simulink model "c09f12_01_avn"  (R2012b)
settings: Solver=ode45  StartTime=0.0  StopTime="(2^(7+2))  * (2^8)"  RelTol=1e-3
undefined symbols (not defined in the file): Down, pfb_coeff_gen_calc, Up, xlipgetpartsetting
libraries: xbsIndex_r4 x7041, casper_library_misc x193, xps_library x58, casper_library_delays x50, simulink x16, dspsigops x12, casper_library_flow_control x5, xbsReplacements_r4 x4, casper_library_ffts_twiddle x2, casper_library_multipliers x2, casper_library_reorder x1
(part 1 of 77)
settings Model: Creator=root  LastModifiedBy=brains
settings DataIOCC: LimitDataPoints=off  SignalLoggingSaveFormat=ModelDataLogs
settings DebuggingCC: FcnCallInpInsideContextMsg=UseLocalSettings  StrictBusMsg=Warning
settings GRTTargetCC: CombineOutputUpdateFcns=off  GRTInterface=on

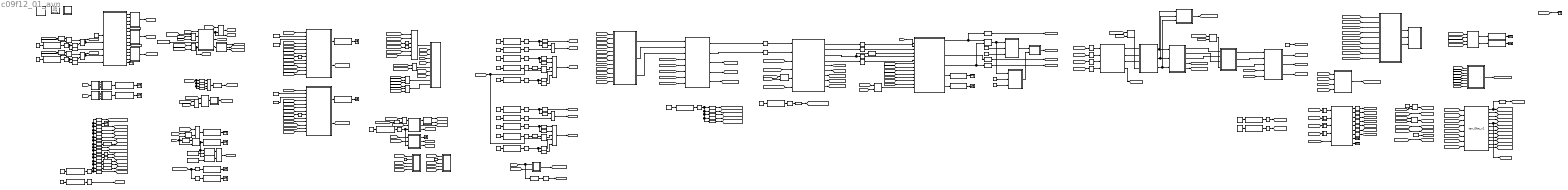
== system c09f12_01_avn ==
  note: Accept 32 data words from ibob,
      | plus a 1 word header,
      | creating UDP packets of length 33 x 64 bits.
      | This block generates the destination IP address.
  note: Data in: 18bits real only x 2
  note: RCS:
      |
      | 1. 04-08-2011
      | - Initial revision.
      | 2. 08-08-2011
      | - New snapshots for easier timing.
      | 3. 17-08-2011
      | - Fixed logic around gbe & xaui snaps.
      | 4. 19-08-2011
      | - Updated timing logic from latest wideband build.
      | ...
      | 5. 17-11-2011
      | - New TVG before CT.
      | - New DV gen in fine chan.
      | - Remove delay on sync in packetiser.
      |
      | New packetiser put in, builds, but 10Gbe doesn't
      | work. Why? If the device is too full?
      |
      | Needs coarse vector accumulator.
      |
      | 6. 10-01-2012
      | - 16 x-engines vs 4 seems to solve VACC overflow
      | on the x-engine.
      | 7. 12-01-2012
      | - Move to 4a 8x to for lab work.
      | - Also mux to bypass window before fine FFT.
      | 8. 18-01-2012
      | - Cleaned up fine snap
      | - Delays between blocks in coarse channelisaiton.
      | 9. 10-02-2012
      | - See subversion for notes.
      | 10. 13-02-2012
      | - Half of channel select in the coarse section,
      | moved from fine buffer.
      | - No more mixer, so real PFB and FFT.
  note: The data out of the QDR
      | ct is 64-bit data ready
      | for the packetiser.
  note: * A resync command will cause the sync_gen to stop issuing sync pulses.
      | * It will then ignore the next input trigger (1PPS), while sync is flushed through the DSP pipeline.
      | * It will then lock onto the next trigger (1PPS) and issue a sync.
      | * Need a multiple of (pfb_fir taps*LCM(FFT reorder orders) *fft bins/parallel inputs =)
      | (4 * LCM(2,2,2,9) * 2048 / 4) = 9216) for sync_period for simulation
  note: data alignment infrastructure to
      | align to within one clock cycle
      | using PPS
  note: clock and synchronisation
      | info
  note: Status registers
  note: LEDs
  note: delay tracking and
      | fringe stopping registers
  note: pol0
  note: pol1
  note: Fine delay tracking and
      | fringe stopping
  note: ADC snap blocks
  " System Generator" : xbsIndex_r4/ System Generator  Tag=genX  xilinxfamily=virtex5  part=xc5vsx95t  speed=-1  package=ff1136  synthesis_tool=XST  clock_wrapper=Clock Enables  directory=./c09f12_01_avn/sysgen  proj_type=Project Navigator  Synth_file=XST Defaults  Impl_file=ISE Defaults  testbench=off  simulink_period=1  sysclk_period=5  dcm_input_clock_period=100  incr_netlist=off  trim_vbits=Everywhere in SubSystem  dbl_ovrd=According to Block Masks  core_generation=According to Block Masks  run_coregen=off  deprecated_control=off  eval_field=0  block_type=sysgen
      settings: block_version=11.4
  AddSub : xbsIndex_r4/AddSub  mode=Addition  use_carryin=off  use_carryout=off  en=off  latency=1  precision=User Defined  arith_type=Unsigned  n_bits=15  bin_pt=0  quantization=Truncate  overflow=Saturate  dbl_ovrd=off  use_behavioral_HDL=off  hw_selection=DSP48  pipelined=on  block_type=addsub
  AddSub1 : xbsIndex_r4/AddSub  mode=Addition  use_carryin=off  use_carryout=off  en=off  latency=1  precision=User Defined  arith_type=Unsigned  n_bits=15  bin_pt=0  quantization=Truncate  overflow=Saturate  dbl_ovrd=off  use_behavioral_HDL=off  hw_selection=DSP48  pipelined=on  block_type=addsub
  Concat : xbsIndex_r4/Concat  num_inputs=3  dbl_ovrd=off  block_type=concat
      settings: block_version=10.1.3
  Concat1 : xbsIndex_r4/Concat  num_inputs=5  dbl_ovrd=off  block_type=concat
      settings: block_version=10.1.3
  Concat{2,6,9,21} (4 alike) : xbsIndex_r4/Concat  num_inputs=2  dbl_ovrd=off  block_type=concat
      Concat2 settings: block_version=10.1.3
      Concat9 settings: block_version=10.1.3
  Concat22 : xbsIndex_r4/Concat  num_inputs=5  dbl_ovrd=off  block_type=concat
      settings: block_version=10.1.3
  Constant : Constant  SampleTime=1/4
  Constant{1,6,9,11,18,27,33,48} (8 alike) : Constant  Value=0
  Constant{10,13,16,21..22,32} (6 alike) : Constant  Value=8
  Constant14 : xbsIndex_r4/Constant  const=1  gui_display_data_type=Fixed-point  arith_type=Boolean  n_bits=1  bin_pt=0  preci_type=Single  exp_width=8  frac_width=24  explicit_period=on  period=1  equ=P=C  opselect=C  inp2=PCIN>>17  opr=+  inp1=P  carry=CIN  dbl_ovrd=off  block_type=constant
  Constant15 : xbsIndex_r4/Constant  const=1  gui_display_data_type=Fixed-point  arith_type=Boolean  n_bits=1  bin_pt=0  preci_type=Single  exp_width=8  frac_width=24  explicit_period=off  period=1  equ=P=C  opselect=C  inp2=PCIN>>17  opr=+  inp1=P  carry=CIN  dbl_ovrd=off  block_type=constant
      settings: block_version=11.4
  Constant17 : xbsIndex_r4/Constant  const=0  gui_display_data_type=Fixed-point  arith_type=Boolean  n_bits=16  bin_pt=14  preci_type=Single  exp_width=8  frac_width=24  explicit_period=on  period=1  equ=P=C  opselect=C  inp2=PCIN>>17  opr=+  inp1=P  carry=CIN  dbl_ovrd=off  block_type=constant
      settings: block_version=11.4
  Constant20 : xbsIndex_r4/Constant  const=0  gui_display_data_type=Fixed-point  arith_type=Boolean  n_bits=1  bin_pt=0  preci_type=Single  exp_width=8  frac_width=24  explicit_period=on  period=1  equ=P=C  opselect=C  inp2=PCIN>>17  opr=+  inp1=P  carry=CIN  dbl_ovrd=off  block_type=constant
      settings: block_version=11.3
  Constant23 : xbsIndex_r4/Constant  const=1  gui_display_data_type=Fixed-point  arith_type=Boolean  n_bits=1  bin_pt=0  preci_type=Single  exp_width=8  frac_width=24  explicit_period=off  period=1  equ=P=C  opselect=C  inp2=PCIN>>17  opr=+  inp1=P  carry=CIN  dbl_ovrd=off  block_type=constant
      settings: block_version=11.4
  Constant24 : xbsIndex_r4/Constant  const=0  gui_display_data_type=Fixed-point  arith_type=Boolean  n_bits=64  bin_pt=0  preci_type=Single  exp_width=8  frac_width=24  explicit_period=off  period=1  equ=P=C  opselect=C  inp2=PCIN>>17  opr=+  inp1=P  carry=CIN  dbl_ovrd=off  block_type=constant
      settings: block_version=11.4
  Constant25 : Constant  Value=100
  Constant29 : Constant  Value=20
  Constant37 : xbsIndex_r4/Constant  const=800000000/4-1  gui_display_data_type=Fixed-point  arith_type=Unsigned  n_bits=32  bin_pt=0  preci_type=Single  exp_width=8  frac_width=24  explicit_period=on  period=1  equ=P=C  opselect=C  inp2=PCIN>>17  opr=+  inp1=P  carry=CIN  dbl_ovrd=off  block_type=constant
      settings: block_version=11.4
  Constant41 : xbsIndex_r4/Constant  const=0  gui_display_data_type=Fixed-point  arith_type=Unsigned  n_bits=32  bin_pt=0  preci_type=Single  exp_width=8  frac_width=24  explicit_period=off  period=1  equ=P=C  opselect=C  inp2=PCIN>>17  opr=+  inp1=P  carry=CIN  dbl_ovrd=off  block_type=constant
      settings: block_version=11.4
  Constant46 : xbsIndex_r4/Constant  const=0  gui_display_data_type=Fixed-point  arith_type=Boolean  n_bits=64  bin_pt=0  preci_type=Single  exp_width=8  frac_width=24  explicit_period=off  period=1  equ=P=C  opselect=C  inp2=PCIN>>17  opr=+  inp1=P  carry=CIN  dbl_ovrd=off  block_type=constant
      settings: block_version=11.4
  Constant5 : xbsIndex_r4/Constant  const=800000000/4+1  gui_display_data_type=Fixed-point  arith_type=Unsigned  n_bits=32  bin_pt=0  preci_type=Single  exp_width=8  frac_width=24  explicit_period=on  period=1  equ=P=C  opselect=C  inp2=PCIN>>17  opr=+  inp1=P  carry=CIN  dbl_ovrd=off  block_type=constant
      settings: block_version=11.4
  Constant7 : Constant  Value=20
  Constant8 : xbsIndex_r4/Constant  const=0  gui_display_data_type=Fixed-point  arith_type=Unsigned  n_bits=32  bin_pt=0  preci_type=Single  exp_width=8  frac_width=24  explicit_period=off  period=1  equ=P=C  opselect=C  inp2=PCIN>>17  opr=+  inp1=P  carry=CIN  dbl_ovrd=off  block_type=constant
      settings: block_version=11.4
  Counter1 : xbsIndex_r4/Counter  cnt_type=Free Running  cnt_to=Inf  operation=Up  start_count=1  cnt_by_val=1  arith_type=Unsigned  n_bits=32  bin_pt=0  load_pin=off  rst=on  en=off  explicit_period=on  period=1  dbl_ovrd=off  use_behavioral_HDL=off  implementation=Fabric  use_rpm=on  block_type=counter
  Counter3 : xbsIndex_r4/Counter  cnt_type=Free Running  cnt_to=Inf  operation=Up  start_count=0  cnt_by_val=1  arith_type=Unsigned  n_bits=31  bin_pt=0  load_pin=off  rst=on  en=on  explicit_period=on  period=1  dbl_ovrd=off  use_behavioral_HDL=off  implementation=DSP48  use_rpm=on  block_type=counter
  Counter8 : xbsIndex_r4/Counter  cnt_type=Free Running  cnt_to=Inf  operation=Up  start_count=0  cnt_by_val=1  arith_type=Unsigned  n_bits=12  bin_pt=0  load_pin=off  rst=on  en=on  explicit_period=on  period=1  dbl_ovrd=off  use_behavioral_HDL=off  implementation=Fabric  block_type=counter
      settings: block_version=11.4
  Delay{1,8,12..22,24..30,32,35..37,39..46} (32 alike) : xbsIndex_r4/Delay  rst=off  infoeditControl=Selection of Reset will increase slice count due to use of real FFs and instead of SRLs  en=off  latency=1  dbl_ovrd=off  reg_retiming=on  block_type=delay
      Delay13 settings: block_version=11.4
      Delay14 settings: block_version=11.4
      Delay15 settings: block_version=11.4
      Delay16 settings: block_version=11.4
      Delay17 settings: block_version=11.4
      Delay18 settings: block_version=11.4
      Delay19 settings: block_version=11.4
      Delay20 settings: block_version=11.4
      Delay21 settings: block_version=11.4
      Delay22 settings: block_version=11.4
      Delay24 settings: block_version=11.4
      Delay25 settings: block_version=11.4
      Delay26 settings: block_version=11.4
      Delay27 settings: block_version=11.4
      Delay28 settings: block_version=11.4
      Delay29 settings: block_version=11.4
      Delay30 settings: block_version=11.4
      Delay32 settings: block_version=11.4
      Delay35 settings: block_version=11.4
      Delay36 settings: block_version=11.4
      Delay37 settings: block_version=11.4
      Delay39 settings: block_version=11.4
      Delay40 settings: block_version=11.4
      Delay41 settings: block_version=11.4
      Delay42 settings: block_version=11.4
  Delay10 : Subsystem  AncestorBlock=casper_library/Delays/pipeline  mask(pipeline){latency=1}
      mask help:
      | An explicitly laid-out delay line to avoid mapping to SRL16s
      | for use in pipelining to help achieve timing closure.
      mask init:
      | pipeline_init(gcb, 'latency', latency);
      mask Display:
      | port_label('input', 1, 'd');
      | port_label('output', 1, 'q');
      | disp(['Z^-', num2str(latency)]);
  Delay100 : Subsystem  AncestorBlock=casper_library/Delays/pipeline  mask(pipeline){latency=2}
      mask help:
      | An explicitly laid-out delay line to avoid mapping to SRL16s
      | for use in pipelining to help achieve timing closure.
      mask init:
      | pipeline_init(gcb, 'latency', latency);
      mask Display:
      | port_label('input', 1, 'd');
      | port_label('output', 1, 'q');
      | disp(['Z^-', num2str(latency)]);
  Delay11 : Subsystem  AncestorBlock=casper_library/Delays/pipeline  mask(pipeline){latency=1}
      mask help:
      | An explicitly laid-out delay line to avoid mapping to SRL16s
      | for use in pipelining to help achieve timing closure.
      mask init:
      | pipeline_init(gcb, 'latency', latency);
      mask Display:
      | port_label('input', 1, 'd');
      | port_label('output', 1, 'q');
      | disp(['Z^-', num2str(latency)]);
  Delay2 : Subsystem  AncestorBlock=casper_library/Delays/pipeline  mask(pipeline){latency=2}
      mask help:
      | An explicitly laid-out delay line to avoid mapping to SRL16s
      | for use in pipelining to help achieve timing closure.
      mask init:
      | pipeline_init(gcb, 'latency', latency);
      mask Display:
      | port_label('input', 1, 'd');
      | port_label('output', 1, 'q');
      | disp(['Z^-', num2str(latency)]);
  Delay23 : Subsystem  AncestorBlock=casper_library/Delays/pipeline  mask(pipeline){latency=1}
      mask help:
      | An explicitly laid-out delay line to avoid mapping to SRL16s
      | for use in pipelining to help achieve timing closure.
      mask init:
      | pipeline_init(gcb, 'latency', latency);
      mask Display:
      | port_label('input', 1, 'd');
      | port_label('output', 1, 'q');
      | disp(['Z^-', num2str(latency)]);
  Delay3 : Subsystem  AncestorBlock=casper_library/Delays/pipeline  mask(pipeline){latency=1}
      mask help:
      | An explicitly laid-out delay line to avoid mapping to SRL16s
      | for use in pipelining to help achieve timing closure.
      mask init:
      | pipeline_init(gcb, 'latency', latency);
      mask Display:
      | port_label('input', 1, 'd');
      | port_label('output', 1, 'q');
      | disp(['Z^-', num2str(latency)]);
  Delay31 : Subsystem  AncestorBlock=casper_library/Delays/pipeline  mask(pipeline){latency=1}
      mask help:
      | An explicitly laid-out delay line to avoid mapping to SRL16s
      | for use in pipelining to help achieve timing closure.
      mask init:
      | pipeline_init(gcb, 'latency', latency);
      mask Display:
      | port_label('input', 1, 'd');
      | port_label('output', 1, 'q');
      | disp(['Z^-', num2str(latency)]);
  Delay33 : Subsystem  AncestorBlock=casper_library/Delays/pipeline  mask(pipeline){latency=1}
      mask help:
      | An explicitly laid-out delay line to avoid mapping to SRL16s
      | for use in pipelining to help achieve timing closure.
      mask init:
      | pipeline_init(gcb, 'latency', latency);
      mask Display:
      | port_label('input', 1, 'd');
      | port_label('output', 1, 'q');
      | disp(['Z^-', num2str(latency)]);
  Delay34 : Subsystem  AncestorBlock=casper_library/Delays/pipeline  mask(pipeline){latency=1}
      mask help:
      | An explicitly laid-out delay line to avoid mapping to SRL16s
      | for use in pipelining to help achieve timing closure.
      mask init:
      | pipeline_init(gcb, 'latency', latency);
      mask Display:
      | port_label('input', 1, 'd');
      | port_label('output', 1, 'q');
      | disp(['Z^-', num2str(latency)]);
  Delay4 : Subsystem  AncestorBlock=casper_library/Delays/pipeline  mask(pipeline){latency=1}
      mask help:
      | An explicitly laid-out delay line to avoid mapping to SRL16s
      | for use in pipelining to help achieve timing closure.
      mask init:
      | pipeline_init(gcb, 'latency', latency);
      mask Display:
      | port_label('input', 1, 'd');
      | port_label('output', 1, 'q');
      | disp(['Z^-', num2str(latency)]);
  Delay5 : Subsystem  AncestorBlock=casper_library/Delays/pipeline  mask(pipeline){latency=1}
      mask help:
      | An explicitly laid-out delay line to avoid mapping to SRL16s
      | for use in pipelining to help achieve timing closure.
      mask init:
      | pipeline_init(gcb, 'latency', latency);
      mask Display:
      | port_label('input', 1, 'd');
      | port_label('output', 1, 'q');
      | disp(['Z^-', num2str(latency)]);
  Delay6 : xbsIndex_r4/Delay  rst=off  infoeditControl=Selection of Reset will increase slice count due to use of real FFs and instead of SRLs  en=off  latency=1  dbl_ovrd=off  reg_retiming=off  block_type=delay
      settings: block_version=11.4
  Delay7 : Subsystem  AncestorBlock=casper_library/Delays/pipeline  mask(pipeline){latency=1}
      mask help:
      | An explicitly laid-out delay line to avoid mapping to SRL16s
      | for use in pipelining to help achieve timing closure.
      mask init:
      | pipeline_init(gcb, 'latency', latency);
      mask Display:
      | port_label('input', 1, 'd');
      | port_label('output', 1, 'q');
      | disp(['Z^-', num2str(latency)]);
  Delay9 : Subsystem  AncestorBlock=casper_library/Delays/pipeline  mask(pipeline){latency=1}
      mask help:
      | An explicitly laid-out delay line to avoid mapping to SRL16s
      | for use in pipelining to help achieve timing closure.
      mask init:
      | pipeline_init(gcb, 'latency', latency);
      mask Display:
      | port_label('input', 1, 'd');
      | port_label('output', 1, 'q');
      | disp(['Z^-', num2str(latency)]);
  Inverter{,1..6} (7 alike) : xbsIndex_r4/Inverter  en=off  latency=0  dbl_ovrd=off  block_type=inv
      settings: block_version=11.4
  Logical1 : xbsIndex_r4/Logical  logical_function=OR  inputs=4  en=off  latency=0  precision=Full  arith_type=Unsigned  n_bits=16  bin_pt=0  align_bp=on  dbl_ovrd=off  block_type=logical
  Logical10 : xbsIndex_r4/Logical  logical_function=AND  inputs=2  en=off  latency=0  precision=Full  arith_type=Unsigned  n_bits=16  bin_pt=0  align_bp=on  dbl_ovrd=off  block_type=logical
  Logical11 : xbsIndex_r4/Logical  logical_function=AND  inputs=2  en=off  latency=0  precision=Full  arith_type=Unsigned  n_bits=16  bin_pt=0  align_bp=on  dbl_ovrd=off  block_type=logical
  Logical12 : xbsIndex_r4/Logical  logical_function=OR  inputs=3  en=off  latency=1  precision=Full  arith_type=Unsigned  n_bits=16  bin_pt=0  align_bp=on  dbl_ovrd=off  block_type=logical
  Logical{5..6,9,14,21} (5 alike) : xbsIndex_r4/Logical  logical_function=OR  inputs=2  en=off  latency=0  precision=Full  arith_type=Unsigned  n_bits=16  bin_pt=0  align_bp=on  dbl_ovrd=off  block_type=logical
      Logical21 settings: block_version=11.4
  Logical17 : xbsIndex_r4/Logical  logical_function=OR  inputs=3  en=off  latency=1  precision=Full  arith_type=Unsigned  n_bits=16  bin_pt=0  align_bp=on  dbl_ovrd=off  block_type=logical
  Logical2 : xbsIndex_r4/Logical  logical_function=AND  inputs=2  en=off  latency=0  precision=Full  arith_type=Unsigned  n_bits=8  bin_pt=2  align_bp=on  dbl_ovrd=off  block_type=logical
      settings: xl_area=[0, 0, 0, 0, 0, 0, 0]
  Logical3 : xbsIndex_r4/Logical  logical_function=OR  inputs=2  en=off  latency=1  precision=Full  arith_type=Unsigned  n_bits=8  bin_pt=2  align_bp=on  dbl_ovrd=off  block_type=logical
      settings: xl_area=[0, 0, 0, 0, 0, 0, 0]
  Logical4 : xbsIndex_r4/Logical  logical_function=OR  inputs=2  en=off  latency=1  precision=Full  arith_type=Unsigned  n_bits=16  bin_pt=0  align_bp=on  dbl_ovrd=off  block_type=logical
  Logical7 : xbsIndex_r4/Logical  logical_function=OR  inputs=6  en=off  latency=1  precision=Full  arith_type=Unsigned  n_bits=16  bin_pt=0  align_bp=on  dbl_ovrd=off  block_type=logical
  Logical8 : xbsIndex_r4/Logical  logical_function=AND  inputs=2  en=off  latency=0  precision=Full  arith_type=Unsigned  n_bits=16  bin_pt=0  align_bp=on  dbl_ovrd=off  block_type=logical
  Register{1..5,19} (6 alike) : xbsIndex_r4/Register  init=0  rst=off  en=on  dbl_ovrd=off  block_type=register
      Register1 settings: block_version=11.4
      Register2 settings: block_version=11.4
      Register3 settings: block_version=11.4
      Register4 settings: block_version=11.4
      Register5 settings: block_version=11.4
  Relational : xbsIndex_r4/Relational  mode=a>b  en=off  latency=1  dbl_ovrd=off  block_type=relational
  Relational1 : xbsIndex_r4/Relational  mode=a<b  en=off  latency=1  dbl_ovrd=off  block_type=relational
  Slice : xbsIndex_r4/Slice  nbits=32  boolean_output=off  mode=Lower Bit Location + Width  bit1=0  base1=MSB of Input  bit0=0  base0=LSB of Input  dbl_ovrd=off  block_type=slice
  Slice{1..2,4,12,15,73} (6 alike) : xbsIndex_r4/Slice  nbits=16  boolean_output=off  mode=Lower Bit Location + Width  bit1=0  base1=MSB of Input  bit0=0  base0=LSB of Input  dbl_ovrd=off  block_type=slice
      settings: infoedit="Extracts a given range of bits from each input sample and presents it at the output.  The output type is ordinarily unsigned with binary point at zero, but can be Boolean when the slice is one bit wide.<P><P>Hardware notes: In hardware this block costs nothing."  block_version=10.1.3
  Slice{3,7..8,10} (4 alike) : xbsIndex_r4/Slice  nbits=16  boolean_output=off  mode=Lower Bit Location + Width  bit1=0  base1=MSB of Input  bit0=16  base0=LSB of Input  dbl_ovrd=off  block_type=slice
      Slice10 settings: block_version=10.1.3
      Slice3 settings: infoedit="Extracts a given range of bits from each input sample and presents it at the output.  The output type is ordinarily unsigned with binary point at zero, but can be Boolean when the slice is one bit wide.<P><P>Hardware notes: In hardware this block costs nothing."  block_version=10.1.3
      Slice7 settings: block_version=10.1.3
      Slice8 settings: infoedit="Extracts a given range of bits from each input sample and presents it at the output.  The output type is ordinarily unsigned with binary point at zero, but can be Boolean when the slice is one bit wide.<P><P>Hardware notes: In hardware this block costs nothing."  block_version=10.1.3
  Slice{11,13,29,33} (4 alike) : xbsIndex_r4/Slice  nbits=1  boolean_output=on  mode=Upper Bit Location + Width  bit1=0  base1=MSB of Input  bit0=0  base0=LSB of Input  dbl_ovrd=off  block_type=slice
      Slice11 settings: block_version=10.1.3
      Slice13 settings: block_version=10.1.3
  Slice14 : xbsIndex_r4/Slice  nbits=15  boolean_output=off  mode=Lower Bit Location + Width  bit1=0  base1=MSB of Input  bit0=0  base0=LSB of Input  dbl_ovrd=off  block_type=slice
      settings: block_version=10.1.3
  Slice16 : xbsIndex_r4/Slice  nbits=32  boolean_output=off  mode=Lower Bit Location + Width  bit1=0  base1=MSB of Input  bit0=0  base0=LSB of Input  dbl_ovrd=off  block_type=slice
  Slice17 : xbsIndex_r4/Slice  nbits=1  boolean_output=on  mode=Lower Bit Location + Width  bit1=0  base1=MSB of Input  bit0=20  base0=LSB of Input  dbl_ovrd=off  block_type=slice
      settings: block_version=10.1.3
  Slice18 : xbsIndex_r4/Slice  nbits=1  boolean_output=on  mode=Lower Bit Location + Width  bit1=0  base1=MSB of Input  bit0=21  base0=LSB of Input  dbl_ovrd=off  block_type=slice
      settings: block_version=10.1.3
  Slice19 : xbsIndex_r4/Slice  nbits=8 - 1 - 1  boolean_output=off  mode=Lower Bit Location + Width  bit1=0  base1=MSB of Input  bit0=22  base0=LSB of Input  dbl_ovrd=off  block_type=slice
      settings: block_version=10.1.3
  Slice21 : xbsIndex_r4/Slice  nbits=10  boolean_output=off  mode=Lower Bit Location + Width  bit1=0  base1=MSB of Input  bit0=10  base0=LSB of Input  dbl_ovrd=off  block_type=slice
      settings: block_version=10.1.3
  Slice24 : xbsIndex_r4/Slice  nbits=26  boolean_output=off  mode=Lower Bit Location + Width  bit1=0  base1=MSB of Input  bit0=0  base0=LSB of Input  dbl_ovrd=off  block_type=slice
      settings: block_version=10.1.3
  Slice30 : xbsIndex_r4/Slice  nbits=6  boolean_output=off  mode=Lower Bit Location + Width  bit1=0  base1=MSB of Input  bit0=0  base0=LSB of Input  dbl_ovrd=off  block_type=slice
  Slice34 : xbsIndex_r4/Slice  nbits=6  boolean_output=off  mode=Lower Bit Location + Width  bit1=0  base1=MSB of Input  bit0=0  base0=LSB of Input  dbl_ovrd=off  block_type=slice
  Slice35 : xbsIndex_r4/Slice  nbits=1  boolean_output=on  mode=Lower Bit Location + Width  bit1=0  base1=MSB of Input  bit0=3  base0=LSB of Input  dbl_ovrd=off  block_type=slice
  Slice36 : xbsIndex_r4/Slice  nbits=1  boolean_output=on  mode=Lower Bit Location + Width  bit1=0  base1=MSB of Input  bit0=2  base0=LSB of Input  dbl_ovrd=off  block_type=slice
  Slice38 : xbsIndex_r4/Slice  nbits=15  boolean_output=off  mode=Lower Bit Location + Width  bit1=0  base1=MSB of Input  bit0=0  base0=LSB of Input  dbl_ovrd=off  block_type=slice
      settings: block_version=10.1.3
  Slice40 : xbsIndex_r4/Slice  nbits=1  boolean_output=on  mode=Lower Bit Location + Width  bit1=0  base1=MSB of Input  bit0=1  base0=LSB of Input  dbl_ovrd=off  block_type=slice
  Slice45 : xbsIndex_r4/Slice  nbits=1  boolean_output=on  mode=Lower Bit Location + Width  bit1=0  base1=MSB of Input  bit0=0  base0=LSB of Input  dbl_ovrd=off  block_type=slice
  Slice6 : xbsIndex_r4/Slice  nbits=10  boolean_output=off  mode=Lower Bit Location + Width  bit1=0  base1=MSB of Input  bit0=0  base0=LSB of Input  dbl_ovrd=off  block_type=slice
      settings: block_version=10.1.3
  Slice78 : xbsIndex_r4/Slice  nbits=1  boolean_output=on  mode=Lower Bit Location + Width  bit1=0  base1=MSB of Input  bit0=0  base0=LSB of Input  dbl_ovrd=off  block_type=slice
      settings: block_version=10.1.3
  Slice9 : xbsIndex_r4/Slice  nbits=32  boolean_output=off  mode=Lower Bit Location + Width  bit1=0  base1=MSB of Input  bit0=32  base0=LSB of Input  dbl_ovrd=off  block_type=slice
  Subsystem : Subsystem
  Subsystem1 : Subsystem
  Subsystem2 : Subsystem
  Subsystem3 : Subsystem
  Subsystem4 : Subsystem
  Terminator{,1..15,17,25} (18 alike) : Terminator
  XSG core config : xps_library/XSG core config  Tag=xps:xsg  hw_sys=ROACH:sx95t  clk_src=adc0_clk  ROACH_clk_src=adc0_clk  ROACH2_clk_src=adc0_clk  clk_rate=800/4  sample_period=1  synthesis_tool=XST
  a0_fd0 : xps_library/software register  Tag=xps:sw_reg  io_dir=From Processor  arith_type=Unsigned  bitwidth=32  bin_pt=0  sample_period=1  gw_name=c09f12_01_avn_a0_fd0_user_data_out
      link override c09f12_01_a0_fd0_user_data_out: arith_type=Unsigned  n_bits=32  bin_pt=0  period=1
  a0_fd1 : xps_library/software register  Tag=xps:sw_reg  io_dir=From Processor  arith_type=Unsigned  bitwidth=32  bin_pt=0  sample_period=1  gw_name=c09f12_01_avn_a0_fd1_user_data_out
      link override c09f12_01_a0_fd1_user_data_out: arith_type=Unsigned  n_bits=32  bin_pt=0  period=1
  a1_fd0 : xps_library/software register  Tag=xps:sw_reg  io_dir=From Processor  arith_type=Unsigned  bitwidth=32  bin_pt=0  sample_period=1  gw_name=c09f12_01_avn_a1_fd0_user_data_out
      link override c09f12_01_a1_fd0_user_data_out: arith_type=Unsigned  n_bits=32  bin_pt=0  period=1
  a1_fd1 : xps_library/software register  Tag=xps:sw_reg  io_dir=From Processor  arith_type=Unsigned  bitwidth=32  bin_pt=0  sample_period=1  gw_name=c09f12_01_avn_a1_fd1_user_data_out
      link override c09f12_01_a1_fd1_user_data_out: arith_type=Unsigned  n_bits=32  bin_pt=0  period=1
  adc_ctrl0 : xps_library/software register  Tag=xps:sw_reg  io_dir=From Processor  arith_type=Unsigned  bitwidth=32  bin_pt=0  sample_period=1  gw_name=c09f12_01_avn_adc_ctrl0_user_data_out
      link override c09f12_01_adc_ctrl0_user_data_out: arith_type=Unsigned  n_bits=32  bin_pt=0  period=1
  adc_ctrl1 : xps_library/software register  Tag=xps:sw_reg  io_dir=From Processor  arith_type=Unsigned  bitwidth=32  bin_pt=0  sample_period=1  gw_name=c09f12_01_avn_adc_ctrl1_user_data_out
      link override c09f12_01_adc_ctrl1_user_data_out: arith_type=Unsigned  n_bits=32  bin_pt=0  period=1
  adc_snap0 : Subsystem  mask(snapshot){storage=bram, dram_dimm=1, dram_clock=200, nsamples=10, data_width=32, offset=on, circap=on, value=on, use_dsp48=off}
      mask prompts: storage "Storage medium"; dram_dimm "DRAM dimm"; dram_clock "DRAM clock rate"; nsamples "Number of Samples (2^?)"; data_width "Data width"; offset "Start delay support"; circap "Circular capture support"; value "Extra value capture support"; use_dsp48 "Use DSP48s to implement counters"
      mask help:
      | Standard snap block, but with the following optional extras;
      |  1) Optionally delay the fabric trigger by a user-specified number of valids.
      |  2) Capture continuously after a trigger until a stop pulse is received. Data is captured into BRAM continuously, with old data being overwritten until a stop command is received. Then stop capturing when memory is filled. This enables you to get some data before and some data after the stop pulse. Use the 'tr_en_cnt' register to determine where you are in your vector. 'Addr' register's MSb now indicates 'busy capturing'.
      |  3) Optionally capture a value on an input port to a register at the same time as the first data sample.
      |  4) Implement counters using DSP48Es to save resources.
      mask init:
      | snapshot_init(gcb, ...
      |     'storage', storage, ...
      |     'dram_dimm', dram_dimm, ...
      |     'dram_clock', dram_clock, ...
      |     'nsamples', nsamples, ...
      |     'data_width', data_width, ...
      |     'offset', offset, ...
      |     'circap', circap, ...
      |     'value', value, ...
      |     'use_dsp48', use_dsp48);
      mask TypeOptions storage: bram | dram
      mask Callback storage: snapshot_callback();
      mask TypeOptions dram_dimm: 1 | 2 | 3 | 4
      mask TypeOptions dram_clock: 200 | 250 | 266 | 300 | 333
      mask TypeOptions data_width: 8 | 16 | 32 | 64 | 128
  adc_snap1 : Subsystem  mask(snapshot){storage=bram, dram_dimm=1, dram_clock=200, nsamples=10, data_width=32, offset=on, circap=on, value=on, use_dsp48=off}
      mask prompts: storage "Storage medium"; dram_dimm "DRAM dimm"; dram_clock "DRAM clock rate"; nsamples "Number of Samples (2^?)"; data_width "Data width"; offset "Start delay support"; circap "Circular capture support"; value "Extra value capture support"; use_dsp48 "Use DSP48s to implement counters"
      mask help:
      | Standard snap block, but with the following optional extras;
      |  1) Optionally delay the fabric trigger by a user-specified number of valids.
      |  2) Capture continuously after a trigger until a stop pulse is received. Data is captured into BRAM continuously, with old data being overwritten until a stop command is received. Then stop capturing when memory is filled. This enables you to get some data before and some data after the stop pulse. Use the 'tr_en_cnt' register to determine where you are in your vector. 'Addr' register's MSb now indicates 'busy capturing'.
      |  3) Optionally capture a value on an input port to a register at the same time as the first data sample.
      |  4) Implement counters using DSP48Es to save resources.
      mask init: same as c09f12_01_avn/adc_snap0
      mask TypeOptions storage: bram | dram
      mask Callback storage: snapshot_callback();
      mask TypeOptions dram_dimm: 1 | 2 | 3 | 4
      mask TypeOptions dram_clock: 200 | 250 | 266 | 300 | 333
      mask TypeOptions data_width: 8 | 16 | 32 | 64 | 128
  adc_sum_sq0 : xps_library/software register  Tag=xps:sw_reg  io_dir=To Processor  arith_type=Unsigned  bitwidth=32  bin_pt=0  sample_period=1  gw_name=c09f12_01_avn_adc_sum_sq0_user_data_in
      link override convert: arith_type=Unsigned  n_bits=32  bin_pt=0
  adc_sum_sq1 : xps_library/software register  Tag=xps:sw_reg  io_dir=To Processor  arith_type=Unsigned  bitwidth=32  bin_pt=0  sample_period=1  gw_name=c09f12_01_avn_adc_sum_sq1_user_data_in
      link override convert: arith_type=Unsigned  n_bits=32  bin_pt=0
  arm1 : xbsIndex_r4/Slice  nbits=1  boolean_output=on  mode=Lower Bit Location + Width  bit1=0  base1=MSB of Input  bit0=2  base0=LSB of Input  dbl_ovrd=off  block_type=slice
      settings: block_version=10.1.3
  arm10 : xbsIndex_r4/Slice  nbits=1  boolean_output=on  mode=Lower Bit Location + Width  bit1=0  base1=MSB of Input  bit0=10  base0=LSB of Input  dbl_ovrd=off  block_type=slice
      settings: block_version=10.1.3
  arm11 : xbsIndex_r4/Slice  nbits=1  boolean_output=on  mode=Lower Bit Location + Width  bit1=0  base1=MSB of Input  bit0=21  base0=LSB of Input  dbl_ovrd=off  block_type=slice
      settings: block_version=10.1.3
  arm12 : xbsIndex_r4/Slice  nbits=1  boolean_output=on  mode=Lower Bit Location + Width  bit1=0  base1=MSB of Input  bit0=11  base0=LSB of Input  dbl_ovrd=off  block_type=slice
      settings: block_version=10.1.3
  arm13 : xbsIndex_r4/Slice  nbits=1  boolean_output=on  mode=Lower Bit Location + Width  bit1=0  base1=MSB of Input  bit0=24  base0=LSB of Input  dbl_ovrd=off  block_type=slice
      settings: block_version=10.1.3
  arm14 : xbsIndex_r4/Slice  nbits=3  boolean_output=off  mode=Lower Bit Location + Width  bit1=0  base1=MSB of Input  bit0=25  base0=LSB of Input  dbl_ovrd=off  block_type=slice
      settings: block_version=10.1.3
  arm2 : xbsIndex_r4/Slice  nbits=1  boolean_output=on  mode=Lower Bit Location + Width  bit1=0  base1=MSB of Input  bit0=3  base0=LSB of Input  dbl_ovrd=off  block_type=slice
      settings: block_version=10.1.3
  arm3 : xbsIndex_r4/Slice  nbits=1  boolean_output=on  mode=Lower Bit Location + Width  bit1=0  base1=MSB of Input  bit0=16  base0=LSB of Input  dbl_ovrd=off  block_type=slice
      settings: block_version=10.1.3
  arm4 : xbsIndex_r4/Slice  nbits=1  boolean_output=on  mode=Lower Bit Location + Width  bit1=0  base1=MSB of Input  bit0=17  base0=LSB of Input  dbl_ovrd=off  block_type=slice
      settings: block_version=10.1.3
  arm5 : xbsIndex_r4/Slice  nbits=1  boolean_output=on  mode=Lower Bit Location + Width  bit1=0  base1=MSB of Input  bit0=18  base0=LSB of Input  dbl_ovrd=off  block_type=slice
      settings: block_version=10.1.3
  arm6 : xbsIndex_r4/Slice  nbits=1  boolean_output=on  mode=Lower Bit Location + Width  bit1=0  base1=MSB of Input  bit0=19  base0=LSB of Input  dbl_ovrd=off  block_type=slice
      settings: block_version=10.1.3
  arm7 : xbsIndex_r4/Slice  nbits=1  boolean_output=on  mode=Lower Bit Location + Width  bit1=0  base1=MSB of Input  bit0=20  base0=LSB of Input  dbl_ovrd=off  block_type=slice
      settings: block_version=10.1.3
  arm8 : xbsIndex_r4/Slice  nbits=1  boolean_output=on  mode=Lower Bit Location + Width  bit1=0  base1=MSB of Input  bit0=9  base0=LSB of Input  dbl_ovrd=off  block_type=slice
      settings: block_version=10.1.3
  arm9 : xbsIndex_r4/Slice  nbits=1  boolean_output=on  mode=Lower Bit Location + Width  bit1=0  base1=MSB of Input  bit0=8  base0=LSB of Input  dbl_ovrd=off  block_type=slice
      settings: block_version=10.1.3
  board_id : xps_library/software register  Tag=xps:sw_reg  io_dir=From Processor  arith_type=Unsigned  bitwidth=32  bin_pt=0  sample_period=1  gw_name=c09f12_01_avn_board_id_user_data_out
      link override c09f12_01_board_id_user_data_out: arith_type=Unsigned  n_bits=32  bin_pt=0  period=1
  bus_create11 : Subsystem  AncestorBlock=casper_library_flow_control/bus_create  mask(bus_create){inputNum=2}
      mask prompts: inputNum "Number of inputs:"
      mask init:
      | bus_create_init(gcb,...
      |     'inputNum', inputNum);
  bus_create2 : Subsystem  AncestorBlock=casper_library_flow_control/bus_create  mask(bus_create){inputNum=4}
      mask prompts: inputNum "Number of inputs:"
      mask init:
      | bus_create_init(gcb,...
      |     'inputNum', inputNum);
  bus_create7 : Subsystem  AncestorBlock=casper_library_flow_control/bus_create  mask(bus_create){inputNum=4}
      mask prompts: inputNum "Number of inputs:"
      mask init:
      | bus_create_init(gcb,...
      |     'inputNum', inputNum);
  bus_create9 : Subsystem  AncestorBlock=casper_library_flow_control/bus_create  mask(bus_create){inputNum=4}
      mask prompts: inputNum "Number of inputs:"
      mask init:
      | bus_create_init(gcb,...
      |     'inputNum', inputNum);
  bus_expand : Subsystem  AncestorBlock=casper_library_flow_control/bus_expand  mask(bus_expand){mode=divisions of arbitrary size, outputNum=2, outputWidth=[1                                     32], outputBinaryPt=[0                                      0], outputArithmeticType=[2                                      0], outputToWorkspace=off, variablePrefix=out, outputToModelAsWell=on}
      mask prompts: outputNum "Number of outputs:"; outputWidth "Output width:"; outputBinaryPt "Output binary point position:"; outputArithmeticType "Output arithmetic type: (Unsigned=0, Signed=1, Boolean=2)"; outputToWorkspace "Output to workspace?"; variablePrefix "Variable name prefix:"; outputToModelAsWell "Output to model as well?"
      mask help:
      | Expands a 'bus' made using a bus_create or Xilinx
      | concat block.
      | The input will be divided into the specified number
      | of outputs with the specified arithmetic types.
      | Divisions are made from most significant bit.
      mask init:
      | bus_expand_init(gcb,...
      |     'mode', mode, ...
      |     'outputNum', outputNum, ...
      |     'outputWidth', outputWidth, ...
      |     'outputBinaryPt', outputBinaryPt, ...
      |     'outputArithmeticType', outputArithmeticType, ...
      |     'outputToWorkspace', outputToWorkspace, ...
      |     'variablePrefix', variablePrefix, ...
      |     'outputToModelAsWell', outputToModelAsWell);
      settings: AttributesFormatString=2 outputs
      mask TypeOptions mode: divisions of equal size | divisions of arbitrary size
      mask Callback mode: bus_expand_callback();
      mask Callback outputWidth: bus_expand_callback();
      mask Callback outputToWorkspace: bus_expand_callback();
  bus_expand6 : Subsystem  AncestorBlock=casper_library_flow_control/bus_expand  mask(bus_expand){mode=divisions of arbitrary size, outputNum=3, outputWidth=[1                                     32                                     32], outputBinaryPt=[0                                      0                                      0], outputArithmeticType=[2                                      0                                      0], show_format=off, outputToWorkspace=off, variablePrefix=out, outputToModelAsWell=on}
      mask prompts: outputNum "Number of outputs:"; outputWidth "Output width:"; outputBinaryPt "Output binary point position:"; outputArithmeticType "Output arithmetic type: (Unsigned=0, Signed=1, Boolean=2)"; show_format "Print format string?"; outputToWorkspace "Output to workspace?"; variablePrefix "Variable name prefix:"; outputToModelAsWell "Output to model as well?"
      mask help:
      | Expands a 'bus' made using a bus_create or Xilinx
      | concat block.
      | The input will be divided into the specified number
      | of outputs with the specified arithmetic types.
      | Divisions are made from most significant bit.
      mask init:
      | bus_expand_init(gcb,...
      |     'mode', mode, ...
      |     'outputNum', outputNum, ...
      |     'outputWidth', outputWidth, ...
      |     'outputBinaryPt', outputBinaryPt, ...
      |     'outputArithmeticType', outputArithmeticType, ...
      |     'show_format', show_format, ...
      |     'outputToWorkspace', outputToWorkspace, ...
      |     'variablePrefix', variablePrefix, ...
      |     'outputToModelAsWell', outputToModelAsWell);
      settings: AttributesFormatString=3 outputs
      mask TypeOptions mode: divisions of equal size | divisions of arbitrary size
      mask Callback mode: bus_expand_callback();
      mask Callback outputWidth: bus_expand_callback();
      mask Callback outputToWorkspace: bus_expand_callback();
  calc_adc_sum_sq : Subsystem
  calc_adc_sum_sq1 : Subsystem
  cd_local_time : Subsystem
  clk_frequency : xps_library/software register  Tag=xps:sw_reg  io_dir=To Processor  arith_type=Unsigned  bitwidth=32  bin_pt=0  sample_period=1  gw_name=c09f12_01_avn_clk_frequency_user_data_in
      link override convert: arith_type=Unsigned  n_bits=32  bin_pt=0
  coarse : Subsystem  mask{fftShift=1, crs_delay=1, pfb_delay=1, fft_delay=1}
      mask prompts: fftShift "Pre-FFT right-shift:"; crs_delay "Post coarse-delay delay:"; pfb_delay "Post PFB delay:"; fft_delay "Post FFT delay:"
  coarse_ctrl : xps_library/software register  Tag=xps:sw_reg  io_dir=From Processor  arith_type=Unsigned  bitwidth=32  bin_pt=0  sample_period=1  gw_name=c09f12_01_avn_coarse_ctrl_user_data_out
      link override c09f12_01_coarse_ctrl_user_data_out: arith_type=Unsigned  n_bits=32  bin_pt=0  period=1
  coarse_delay : Subsystem
  coarse_delay0 : xps_library/software register  Tag=xps:sw_reg  io_dir=From Processor  arith_type=Unsigned  bitwidth=32  bin_pt=0  sample_period=1  gw_name=c09f12_01_avn_coarse_delay0_user_data_out
      link override c09f12_01_coarse_delay0_user_data_out: arith_type=Unsigned  n_bits=32  bin_pt=0  period=1
  coarse_delay1 : xps_library/software register  Tag=xps:sw_reg  io_dir=From Processor  arith_type=Unsigned  bitwidth=32  bin_pt=0  sample_period=1  gw_name=c09f12_01_avn_coarse_delay1_user_data_out
      link override c09f12_01_coarse_delay1_user_data_out: arith_type=Unsigned  n_bits=32  bin_pt=0  period=1
  control : xps_library/software register  Tag=xps:sw_reg  io_dir=From Processor  arith_type=Unsigned  bitwidth=32  bin_pt=0  sample_period=1  gw_name=c09f12_01_avn_control_user_data_out
      link override c09f12_01_control_user_data_out: arith_type=Unsigned  n_bits=32  bin_pt=0  period=1
  convert : Subsystem
  ct_tvg : Subsystem  mask{fine_bits=12, mux_latency=2}
      mask prompts: fine_bits "Fine channels (2^?):"; mux_latency "Mux latency:"
  decat0 : Subsystem
  decat1 : Subsystem
  delay_tr_status0 : Subsystem  Tag=xps:sw_reg  mask{io_dir=To Processor, arith_type=Unsigned, bitwidth=32, bin_pt=0, sample_period=1, latency=0}
      link override convert: arith_type=Unsigned  n_bits=32  bin_pt=0
      mask prompts: io_dir "I/O direction"; arith_type "Data Type"; bitwidth "Data bitwidth"; bin_pt "Data binary point"; sample_period "Sample period"
      mask init:
      | gw_name = clear_name(gcb);
      | config.source = str2func('software_register_init');
      | config.toplevel = gcb;
      | xBlock( config, {io_dir, arith_type, bitwidth, bin_pt, ... 
      |     sample_period, gw_name, latency});
      mask TypeOptions io_dir: From Processor | To Processor
      mask TypeOptions arith_type: Unsigned | Signed  (2's comp)
  delay_tr_status1 : Subsystem  Tag=xps:sw_reg  mask{io_dir=To Processor, arith_type=Unsigned, bitwidth=32, bin_pt=0, sample_period=1, latency=0}
      link override convert: arith_type=Unsigned  n_bits=32  bin_pt=0
      mask prompts: io_dir "I/O direction"; arith_type "Data Type"; bitwidth "Data bitwidth"; bin_pt "Data binary point"; sample_period "Sample period"
      mask init:
      | gw_name = clear_name(gcb);
      | config.source = str2func('software_register_init');
      | config.toplevel = gcb;
      | xBlock( config, {io_dir, arith_type, bitwidth, bin_pt, ... 
      |     sample_period, gw_name, latency});
      mask TypeOptions io_dir: From Processor | To Processor
      mask TypeOptions arith_type: Unsigned | Signed  (2's comp)
  edge_detect{1,3..7} (6 alike) : casper_library_misc/edge_detect  edge=Rising  polarity=Active High  x_in=[0 0.08 0.08 0.16 0.16 0.24 0.24 0.32 0.32 0.4]  y_in="[-1 -1  1  1  1  1  1  1  1  1]"  x_out=[0.6 0.68 0.68 0.76 0.76 0.84 0.84 0.92 0.92 1]  y_out="[-1 -1  1  1 -1 -1 -1 -1 -1 -1]"
  edge_detect2 : Subsystem  AncestorBlock=casper_library_misc/edge_detect  mask(edge_detect){edge=Falling, polarity=Active High, x_in=[0 0.08 0.08 0.16 0.16 0.24 0.24 0.32 0.32 0.4], y_in=[1  1 -1 -1 -1 -1 -1 -1 -1 -1], x_out=[0.6 0.68 0.68 0.76 0.76 0.84 0.84 0.92 0.92 1], y_out=[-1 -1  1  1 -1 -1 -1 -1 -1 -1]}
      mask prompts: edge "Edge Type"; polarity "Output Polarity"; x_in "Input X Positions"; y_in "Input Y Positions"; x_out "Output X Positions"; y_out "Output Y Positions"
      mask help: Output is active for one-cycle after each edge of the specified type (i.e. rising, falling or both).
      mask init:
      | edge_detect_init(gcb,...
      |     'edge',edge,...
      |     'polarity',polarity,...
      |     'x_in',x_in,...
      |     'x_out',x_out,...
      |     'y_in',y_in,...
      |     'y_out',y_out);
      | 
      | x_in_num=str2num(getfield(getfield(get_param(gcb,'UserData'),'parameters'),'x_in'));
      | x_out_num=str2num(getfield(getfield(get_param(gcb,'UserData'),'parameters'),'x_out'));
      | y_in_num=str2num(getfield(getfield(get_param(gcb,'UserData'),'parameters'),'y_in'));
      | y_out_num=str2num(getfield(getfield(get_param(gcb,'UserData'),'parameters'),'y_out'));
      settings: AttributesFormatString=|
      | falling edges
      | active high
      mask Help: Output is active for one-cycle after each edge of the specified type (i.e. rising, falling, or both).  Latency is zero.
      mask TypeOptions edge: Rising | Falling | Both
      mask TypeOptions polarity: Active High | Active Low
      mask Display:
      | plot(x_in_num,0.5+y_in_num*0.2);
      | plot(x_out_num,0.5+y_out_num*0.2);
  eq0 : Subsystem  Tag=xps:bram  AncestorBlock=xps_library/Shared BRAM  mask{arith_type=Unsigned, addr_width=12, data_width=32, reg_prim_output=on, reg_core_output=on, optimization=Minimum_Area, data_bin_pt=0, init_vals=[0:2^10-1], sample_rate=1}
      mask prompts: arith_type "Output Data Type"; addr_width "Address width"; data_width "Data Width"; reg_prim_output "Register Primitive Output"; reg_core_output "Register Core Output"; data_bin_pt "Data Binary Point"; init_vals "Initial 32-bit values (simulation only)"; sample_rate "Sample rate"
      mask init:
      | shared_bram_mask;
      mask TypeOptions arith_type: Unsigned | Signed  (2's comp)
      mask TypeOptions data_width: 8 | 16 | 32 | 64 | 128
      mask TypeOptions optimization: Minimum_Area | Low_Power
  eq1 : Subsystem  Tag=xps:bram  AncestorBlock=xps_library/Shared BRAM  mask{arith_type=Unsigned, addr_width=12, data_width=32, reg_prim_output=on, reg_core_output=on, optimization=Minimum_Area, data_bin_pt=0, init_vals=[0:2^10-1], sample_rate=1}
      mask prompts: arith_type "Output Data Type"; addr_width "Address width"; data_width "Data Width"; reg_prim_output "Register Primitive Output"; reg_core_output "Register Core Output"; data_bin_pt "Data Binary Point"; init_vals "Initial 32-bit values (simulation only)"; sample_rate "Sample rate"
      mask init:
      | shared_bram_mask;
      mask TypeOptions arith_type: Unsigned | Signed  (2's comp)
      mask TypeOptions data_width: 8 | 16 | 32 | 64 | 128
      mask TypeOptions optimization: Minimum_Area | Low_Power
  err_clear_sim3 : Constant  Value=0
  err_clear_sim4 : Constant  Value=0
  fdfs : Subsystem  mask{coarse_fft_bits=9, fine_fft_bits=12, data_bits=18 + 12 + 1, data_bp=17}
      mask prompts: coarse_fft_bits "Coarse FFT points (2^?):"; fine_fft_bits "Fine FFT points (2^?):"; data_bits "Input bits:"; data_bp "Input binary pt:"
      mask init:
      | set_param([gcb, '/expand_data_in'], 'outputWidth', 'data_bits*2');
      | set_param([gcb, '/expand_fd0'], ...
      |     'outputWidth', '[1 (data_bits*2) 1 1 (coarse_fft_bits-1+fine_fft_bits)]', ...
      |     'outputBinaryPt', '[0 0 0 0 0]', ...
      |     'outputArithmeticType', '[2 0 2 2 0]');
      | set_param([gcb, '/fd_fs_tvg0/exp_data'], ...
      |     'outputWidth', '[(data_bits*2) (1+1+(coarse_fft_bits-1+fine_fft_bits))]', ...
      |     'outputBinaryPt', '[0 0]', ...
      |     'outputArithmeticType', '[0 0]');
  fine : Subsystem  mask{coarse_chan_bits=8, parallel_coarse_streams=1, fine_fft_bits=12}
      mask prompts: coarse_chan_bits "Coarse FFT channels (2^?):"; parallel_coarse_streams "Parallel coarse streams (2^?):"; fine_fft_bits "Fine FFT points (2^?):"
  fine_ctrl : xps_library/software register  Tag=xps:sw_reg  io_dir=From Processor  arith_type=Unsigned  bitwidth=32  bin_pt=0  sample_period=1  gw_name=c09f12_01_avn_fine_ctrl_user_data_out
      link override c09f12_01_fine_ctrl_user_data_out: arith_type=Unsigned  n_bits=32  bin_pt=0  period=1
  fstatcbits0 : xbsIndex_r4/Constant  const=9  gui_display_data_type=Fixed-point  arith_type=Unsigned  n_bits=5  bin_pt=0  preci_type=Single  exp_width=8  frac_width=24  explicit_period=off  period=1  equ=P=C  opselect=C  inp2=PCIN>>17  opr=+  inp1=P  carry=CIN  dbl_ovrd=off  block_type=constant
      settings: block_version=11.4
  fstatcbits1 : xbsIndex_r4/Constant  const=9  gui_display_data_type=Fixed-point  arith_type=Unsigned  n_bits=5  bin_pt=0  preci_type=Single  exp_width=8  frac_width=24  explicit_period=off  period=1  equ=P=C  opselect=C  inp2=PCIN>>17  opr=+  inp1=P  carry=CIN  dbl_ovrd=off  block_type=constant
      settings: block_version=11.4
  fstatfbits0 : xbsIndex_r4/Constant  const=12  gui_display_data_type=Fixed-point  arith_type=Unsigned  n_bits=5  bin_pt=0  preci_type=Single  exp_width=8  frac_width=24  explicit_period=off  period=1  equ=P=C  opselect=C  inp2=PCIN>>17  opr=+  inp1=P  carry=CIN  dbl_ovrd=off  block_type=constant
      settings: block_version=11.4
  fstatfbits1 : xbsIndex_r4/Constant  const=12  gui_display_data_type=Fixed-point  arith_type=Unsigned  n_bits=5  bin_pt=0  preci_type=Single  exp_width=8  frac_width=24  explicit_period=off  period=1  equ=P=C  opselect=C  inp2=PCIN>>17  opr=+  inp1=P  carry=CIN  dbl_ovrd=off  block_type=constant
      settings: block_version=11.4
  fstatus0 : xps_library/software register  Tag=xps:sw_reg  io_dir=To Processor  arith_type=Unsigned  bitwidth=32  bin_pt=0  sample_period=1  gw_name=c09f12_01_avn_fstatus0_user_data_in
      link override convert: arith_type=Unsigned  n_bits=32  bin_pt=0
  fstatus1 : xps_library/software register  Tag=xps:sw_reg  io_dir=To Processor  arith_type=Unsigned  bitwidth=32  bin_pt=0  sample_period=1  gw_name=c09f12_01_avn_fstatus1_user_data_in
      link override convert: arith_type=Unsigned  n_bits=32  bin_pt=0
  gbe0 : xps_library/ten_Gbe_v2  Tag=xps:tengbe_v2  flavour=cx4  slot=1  port_r1=0  port_r2_cx4=0  port_r2_sfpp=0  rx_dist_ram=on  large_frames=off  show_param=on  pre_emph_r2=0.74  pre_emph=3  post_emph_r2=0.18  rxeqmix_r2=7  swing_r2=940  swing=800  fab_en=off  fab_mac=hex2dec('123456780000')  fab_ip=192*(2^24) + 168*(2^16) + 5*(2^8) + 20*(2^0)  fab_udp=10000  fab_gate=1  cpu_rx_en=on  cpu_tx_en=on
  gbe_err : Subsystem  mask{payload_len=32}
      mask prompts: payload_len "Packet payload length in 64-bit words?"
      mask init:
      | packet_len = payload_len + 1;
      | packet_bits = ceil(log2(packet_len));
      | payload_bits = ceil(log2(payload_len));
  gbe_ip0 : xps_library/software register  Tag=xps:sw_reg  io_dir=From Processor  arith_type=Unsigned  bitwidth=32  bin_pt=0  sample_period=1  gw_name=c09f12_01_avn_gbe_ip0_user_data_out
      link override c09f12_01_gbe_ip0_user_data_out: arith_type=Unsigned  n_bits=32  bin_pt=0  period=1
  gbe_port : xps_library/software register  Tag=xps:sw_reg  io_dir=From Processor  arith_type=Unsigned  bitwidth=32  bin_pt=0  sample_period=1  gw_name=c09f12_01_avn_gbe_port_user_data_out
      link override c09f12_01_gbe_port_user_data_out: arith_type=Unsigned  n_bits=32  bin_pt=0  period=1
  gbe_tx_cnt0 : xps_library/software register  Tag=xps:sw_reg  io_dir=To Processor  arith_type=Unsigned  bitwidth=32  bin_pt=0  sample_period=1  gw_name=c09f12_01_avn_gbe_tx_cnt0_user_data_in
      link override convert: arith_type=Unsigned  n_bits=32  bin_pt=0
  gbe_tx_err_cnt0 : xps_library/software register  Tag=xps:sw_reg  io_dir=To Processor  arith_type=Unsigned  bitwidth=32  bin_pt=0  sample_period=1  gw_name=c09f12_01_avn_gbe_tx_err_cnt0_user_data_in
      link override convert: arith_type=Unsigned  n_bits=32  bin_pt=0
  katadc0 : Subsystem  Tag=xps:katadc  AncestorBlock=xps_library/katadc  mask(katadc){adc_brd=adc0, adc_interleave=off, bypass_auto=off, en_gain=on, adc_clk_rate=800, sample_period=1}
      mask prompts: adc_brd "ADC board"; adc_interleave "ADC interleave mode"; bypass_auto "Bypass auto config"; en_gain "Enable gain"; adc_clk_rate "ADC sampling rate (MHz)"; sample_period "Sample period"
      mask init:
      | name = [gcs, get_param(gcb, 'Name')];
      | katadc_init(gcb, ...
      |     'name', name, ...
      |     'adc_brd', adc_brd, ...
      |     'adc_interleave', adc_interleave, ...
      |     'bypass_auto', bypass_auto, ...
      |     'en_gain', en_gain, ...
      |     'adc_clk_rate', adc_clk_rate, ...
      |     'sample_period', sample_period);
      mask TypeOptions adc_brd: adc0 | adc1
  ld_time_lsw0 : xps_library/software register  Tag=xps:sw_reg  io_dir=From Processor  arith_type=Unsigned  bitwidth=32  bin_pt=0  sample_period=1  gw_name=c09f12_01_avn_ld_time_lsw0_user_data_out
      link override c09f12_01_ld_time_lsw0_user_data_out: arith_type=Unsigned  n_bits=32  bin_pt=0  period=1
  ld_time_lsw1 : xps_library/software register  Tag=xps:sw_reg  io_dir=From Processor  arith_type=Unsigned  bitwidth=32  bin_pt=0  sample_period=1  gw_name=c09f12_01_avn_ld_time_lsw1_user_data_out
      link override c09f12_01_ld_time_lsw1_user_data_out: arith_type=Unsigned  n_bits=32  bin_pt=0  period=1
  ld_time_msw0 : xps_library/software register  Tag=xps:sw_reg  io_dir=From Processor  arith_type=Unsigned  bitwidth=32  bin_pt=0  sample_period=1  gw_name=c09f12_01_avn_ld_time_msw0_user_data_out
      link override c09f12_01_ld_time_msw0_user_data_out: arith_type=Unsigned  n_bits=32  bin_pt=0  period=1
  ld_time_msw1 : xps_library/software register  Tag=xps:sw_reg  io_dir=From Processor  arith_type=Unsigned  bitwidth=32  bin_pt=0  sample_period=1  gw_name=c09f12_01_avn_ld_time_msw1_user_data_out
      link override c09f12_01_ld_time_msw1_user_data_out: arith_type=Unsigned  n_bits=32  bin_pt=0  period=1
  leds : Subsystem
  man_sync1 : xbsIndex_r4/Slice  nbits=1  boolean_output=on  mode=Lower Bit Location + Width  bit1=0  base1=MSB of Input  bit0=1  base0=LSB of Input  dbl_ovrd=off  block_type=slice
      settings: block_version=10.1.3
  mcount_lsw : xps_library/software register  Tag=xps:sw_reg  io_dir=To Processor  arith_type=Unsigned  bitwidth=32  bin_pt=0  sample_period=1  gw_name=c09f12_01_avn_mcount_lsw_user_data_in
      link override convert: arith_type=Unsigned  n_bits=32  bin_pt=0
  mcount_msw : xps_library/software register  Tag=xps:sw_reg  io_dir=To Processor  arith_type=Unsigned  bitwidth=32  bin_pt=0  sample_period=1  gw_name=c09f12_01_avn_mcount_msw_user_data_in
      link override convert: arith_type=Unsigned  n_bits=32  bin_pt=0
  packetiser : Subsystem  mask{payload_bits=7-2, num_headers=1, x_bits=4, freq_bits=12}
      mask prompts: payload_bits "Payload length(2^?):"; num_headers "Expected headers:"; x_bits "X-engines (2^?):"; freq_bits "Fine channels (2^?):"
  packetiser_tvg_contiguous : Subsystem  mask{payload_bits=7-2, fft_bits=12, xeng_bits=4}
      mask prompts: payload_bits "packet size (2^? 64 bit words)"; fft_bits "fft_size (2^?)"; xeng_bits "x_engines (2^?)"
  pps_count : xps_library/software register  Tag=xps:sw_reg  io_dir=To Processor  arith_type=Unsigned  bitwidth=32  bin_pt=0  sample_period=1  gw_name=c09f12_01_avn_pps_count_user_data_in
      link override convert: arith_type=Unsigned  n_bits=32  bin_pt=0
  qdr_ct : Subsystem  mask{idepth=12, odepth=7, which_qdr=qdr0, swap_input=yes, output_order=interleaved, step_bits=12-4, custom_map=[0 2 4 6 8 10 12 14 1 3 5 7 9 11 13 15]}
      mask prompts: idepth "Input vector length (2^?)"; odepth "Output vector length (2^?)"; which_qdr "QDR SRAM chip"; swap_input "Swap input halves?"; output_order "Output column order"; step_bits "Interleave step (2^?)"; custom_map "Custom map"
      mask help:
      | Writes vectors in as rows in matrix and reads
      | out columns. Order in which columns read out
      | determined by 'Output column order' parameter.
      mask init:
      | if strcmp(output_order, 'interleaved') == 1 && (step_bits > idepth-1) ,
      |     disp('Can''t make step size bigger than (output vector bit size - 1)')
      |     return;
      | end    
      | 
      | if strcmp(output_order, 'custom') && (...
      |         length(unique(custom_map)) ~= 2^idepth ||...
      |         ~isempty(find(custom_map < 0)) || ...
      |         ~isempty(find(custom_map > (2^idepth)-1))),
      |     disp('Custom map elements must be unique in range 0->2^(input vector)-1');
      |     return;
      | end
      | 
      | % set up output order (in order, interleaved, or custom)
      | map = 0 : (2^idepth)-1;
      | if strcmp(swap_input, 'yes'),
      |     map = [map((length(map)/2)+1:end), map(1:length(map)/2)];
      | end
      | if strcmp(output_order, 'interleaved'),
      |     index = zeros(1, 2^idepth);
      |     step_size = 2^(idepth-step_bits);
      |     for ctr = 0:(2^step_bits)-1,
      |         start = (ctr * step_size) + 1;
      |         finish = start + step_size - 1;
      |         index(start:finish) = ctr+1 : 2^step_bits : 2^idepth;
      |     end
      |     map = map(index);
      |     clear index;
      | elseif strcmp(output_order, 'custom'),
      |     map = custom_map;
      | end
      | 
      | %generate map so that two samples from same position in 
      | %subsequent input vectors are written into same address
      | map = reshape([map; 2^idepth+map],1 ,2^(idepth+1));
      | 
      | set_param([gcb, '/reorder'], ...
      |     'map', ['[',num2str(map),']']);
      | set_param([gcb, '/qdr'], 'which_qdr', which_qdr);
      mask TypeOptions which_qdr: qdr0 | qdr1
      mask TypeOptions swap_input: no | yes
      mask TypeOptions output_order: in order | interleaved | custom
  quantisation : Subsystem  mask{fineChanBits=12, dataInBits=18 + 12 + 1, dataInBinaryPt=17, coeffsBits=16, coeffsBinaryPt=1, dataOutBits=4, dataOutBinaryPt=3, initialValue=4}
      mask prompts: fineChanBits "Fine channels (2^?):"; dataInBits "Data in, width:"; dataInBinaryPt "Data in, binary pt:"; coeffsBits "Coeffs, width:"; coeffsBinaryPt "Coeffs, binary pt:"; dataOutBits "Data out, width:"; dataOutBinaryPt "Data out, binary pt:"; initialValue "Initial value:"
      mask init:
      | set_param([gcb, '/expand_data_in'], 'outputWidth', 'dataInBits*2');
  rcs : Subsystem  AncestorBlock=casper_library_misc/rcs  mask(rcs){app_src=timestamp, lib_src=timestamp, user_val=1}
      mask prompts: app_src "Application revision info to capture"; lib_src "CASPER libraries revision info to capture"; user_val "User specified value"
      mask help:
      | Embeds revision control information for the user design and libraries.
      | On failure to locate specified revision information, falls back to
      | timestamps (current time for libraries).
      | A user specified value is also stored.
      mask init:
      | rcs_init(gcb, ...
      |     'app_src', app_src, ...
      |     'lib_src', lib_src);
      mask TypeOptions app_src: timestamp | git | svn
      mask TypeOptions lib_src: timestamp | git | svn
  repack_for_snap : Subsystem
  snap_debug : Subsystem  AncestorBlock=casper_library_scopes/snapshot  mask(snapshot){storage=bram, dram_dimm=1, dram_clock=200, nsamples=10, data_width=128, offset=on, circap=off, value=off, use_dsp48=on}
      mask prompts: storage "Storage medium"; dram_dimm "DRAM dimm"; dram_clock "DRAM clock rate"; nsamples "Number of Samples (2^?)"; data_width "Data width"; offset "Start delay support"; circap "Circular capture support"; value "Extra value capture support"; use_dsp48 "Use DSP48s to implement counters"
      mask help:
      | Standard snap block, but with the following optional extras;
      |  1) Optionally delay the fabric trigger by a user-specified number of valids.
      |  2) Capture continuously after a trigger until a stop pulse is received. Data is captured into BRAM continuously, with old data being overwritten until a stop command is received. Then stop capturing when memory is filled. This enables you to get some data before and some data after the stop pulse. Use the 'tr_en_cnt' register to determine where you are in your vector. 'Addr' register's MSb now indicates 'busy capturing'.
      |  3) Optionally capture a value on an input port to a register at the same time as the first data sample.
      |  4) Implement counters using DSP48Es to save resources.
      mask init: same as c09f12_01_avn/adc_snap0
      mask TypeOptions storage: bram | dram
      mask Callback storage: snapshot_callback();
      mask TypeOptions dram_dimm: 1 | 2 | 3 | 4
      mask TypeOptions dram_clock: 200 | 250 | 266 | 300 | 333
      mask TypeOptions data_width: 8 | 16 | 32 | 64 | 128
  sync_period_constant : xbsIndex_r4/Constant  const=2 * 2 * 2^9 * 2^12 * 2^7 / 2  gui_display_data_type=Fixed-point  arith_type=Unsigned  n_bits=31  bin_pt=0  preci_type=Single  exp_width=8  frac_width=24  explicit_period=off  period=1  equ=P=C  opselect=C  inp2=PCIN>>17  opr=+  inp1=P  carry=CIN  dbl_ovrd=off  block_type=constant
  timing : Subsystem  mask{reset_period=5, sync_gen_bits=31}
      mask prompts: reset_period "Master reset time (sync pulses)"; sync_gen_bits "Size of sync generator counter (bits)"
  trig0 : Subsystem  mask{mult_latency=3}
      mask prompts: mult_latency "Multiplier latency"
  trig1 : Subsystem  mask{mult_latency=3}
      mask prompts: mult_latency "Multiplier latency"
  trig_level : xps_library/software register  Tag=xps:sw_reg  io_dir=From Processor  arith_type=Unsigned  bitwidth=32  bin_pt=0  sample_period=1  gw_name=c09f12_01_avn_trig_level_user_data_out
      link override c09f12_01_trig_level_user_data_out: arith_type=Unsigned  n_bits=32  bin_pt=0  period=1
  xaui_pack0 : Subsystem  mask{payload_len=32, xeng_bits=2, chan_bits=12, skip_xeng_bits=2}
      mask prompts: payload_len "Payload Length (in 64 bit words)"; xeng_bits "Number of X engines (2^?)"; chan_bits "Number of Frequency channels (2^?)"; skip_xeng_bits "X engines per IP address (2^?)"
      mask help: Packetizes data coming in over a XAUI interface. A packet consists of a 64 bit header (48 bits of "mcnt" and 16 bits of antenna), followed by 64 x "payload" bits of payload. "Mcnt" (master count) is a counter which keeps track of how many packets have been transmitted since the last "mrst".
      mask init:
      | packet_len = payload_len + 1;
      | packet_bits = ceil(log2(packet_len));
      | payload_bits = ceil(log2(payload_len));
  wires:
  coarse/1(sync_out) -> Delay22/1
  [coarse_chan_select] -> fine/3(coarse_chan_sel)
  Constant9/1 -> coarse_ctrl/1
  coarse_ctrl/1 -> Delay17/1
  Slice6/1 -> [coarse_fft_shift]
  [coarse_fft_shift] -> coarse/4(fft_shift)
  Constant18/1 -> control/1
  control/1 -> Delay41/1
  Slice78/1 -> [sys_rst]
  man_sync1/1 -> edge_detect7/1
  edge_detect7/1 -> [man_sync]
  arm1/1 -> edge_detect6/1
  edge_detect6/1 -> [arm]
  arm2/1 -> edge_detect5/1
  edge_detect5/1 -> [clr_status]
  arm3/1 -> edge_detect4/1
  edge_detect4/1 -> [tvg_en]
  arm4/1 -> [ct_tvg]
  arm5/1 -> [packetiser_tvg]
  arm6/1 -> [fd_fs_tvg]
  arm7/1 -> [adc_tvg]
  arm8/1 -> Delay100/1(d)
  arm9/1 -> Delay2/1(d)
  Delay100/1(q) -> [gbe_enable]
  Delay2/1(q) -> [gbe_rst]
  Constant1/1 -> board_id/1
  board_id/1 -> Delay42/1
  coarse/3(fft_of0) -> [crs_fft_or0]
  Counter8/1 -> eq1/1(addr), eq0/1(addr)
  Constant41/1 -> eq0/2(data_in)
  Constant46/1 -> eq0/3(we)
  [eq0_coeffs] -> Delay46/1
  fine/5(fft_or0) -> [fine_fft_or0]
  coarse/2(data_out) -> Delay24/1
  Delay8/1 -> [eq0_data]
  [eq0_data] -> Delay44/1
  Delay1/1 -> [eq0_sync]
  [eq0_sync] -> Delay43/1
  [sync] -> Terminator2/1
  quantisation/4(quant_of) -> [quant_or]
  fstatus0/1 -> Terminator9/1
  Subsystem/1(status) -> fstatus0/1
  Constant6/1 -> fine_ctrl/1
  [fine_fft_shift] -> fine/4(fine_fft_shift)
  [mrst] -> packetiser/4(mrst)
  [board_id] -> packetiser/5(antbase)
  xaui_pack0/6(sync) -> Delay31/1(d)
  xaui_pack0/7(mrst) -> Delay34/1(d)
  xaui_pack0/5(discard) -> Delay33/1(d)
  [gbe_base_ip] -> xaui_pack0/5(base_ip)
  xaui_pack0/1(dout) -> Delay9/1(d)
  xaui_pack0/2(valid_out) -> Delay23/1(d)
  xaui_pack0/3(dest_ip) -> Delay10/1(d)
  xaui_pack0/4(eof) -> Delay11/1(d)
  Delay3/1(q) -> xaui_pack0/1(din)
  Delay4/1(q) -> xaui_pack0/2(oob)
  Delay5/1(q) -> xaui_pack0/3(valid_in)
  Delay7/1(q) -> xaui_pack0/4(linkdown_in)
  Delay31/1(q) -> [xaui_sync]
  Delay33/1(q) -> [xaui_pkt_err]
  Delay34/1(q) -> [xaui_mrst]
  [gbe_enable] -> Logical2/2
  xaui_pack0/8(hdr) -> Terminator11/1
  xaui_pack0/9(hdr_valid) -> Terminator10/1
  [xaui_data] -> Delay3/1(d)
  [xaui_oob] -> Delay4/1(d)
  [xaui_valid] -> Delay5/1(d)
  [xaui_link_dn] -> Delay7/1(d)
  Delay9/1(q) -> [xaui_pkt_data]
  Delay23/1(q) -> [xaui_pkt_valid]
  Delay10/1(q) -> [xaui_pkt_ip]
  Delay11/1(q) -> [xaui_pkt_eof]
  [xaui_pkt_valid] -> Logical2/1
  Logical3/1 -> [gbe_rst_int]
  [gbe_rst] -> Logical3/2
  Constant20/1 -> Logical3/1
  Logical2/1 -> [gbe_txvld]
  [xaui_pkt_data] -> [gbe_txd]
  [xaui_pkt_ip] -> [gbe_txip]
  [xaui_pkt_eof] -> [gbe_txeof]
  [xaui_pkt_err] -> [gbe_tx_discard]
  [gbe_rst_int] -> gbe0/1
  [gbe_txd] -> gbe0/2
  [gbe_txvld] -> gbe0/3
  [gbe_txip] -> gbe0/4
  [gbe_txport] -> gbe0/5
  [gbe_txeof] -> gbe0/6
  [gbe_rxack] -> gbe0/7
  Constant14/1 -> [gbe_rxack]
  [gbe_rxack] -> gbe0/8
  Constant17/1 -> [xaui_link_dn]
  gbe_err/1(tx_cnt) -> gbe_tx_cnt0/1
  [clr_status] -> gbe_err/1(rst)
  gbe_err/2(err_cnt) -> gbe_tx_err_cnt0/1
  gbe_tx_cnt0/1 -> Terminator7/1
  gbe_tx_err_cnt0/1 -> Terminator8/1
  [gbe_tx_discard] -> gbe_err/2(discard)
  [gbe_txeof] -> gbe_err/3(eof)
  [gbe_txvld] -> gbe_err/4(valid)
  [tvg_en] -> Register1/2
  [packetiser_tvg] -> Register1/1
  packetiser/1(out_pkt) -> [xaui_data]
  Inverter/1 -> [gbe_ldn0]
  gbe0/1 -> [gbe_up], Inverter/1
  gbe0/2 -> [gbe_rx]
  gbe0/3 -> [gbe_tx]
  gbe0/4 -> [gbe_tx_full]
  gbe0/5 -> [gbe_tx_over], [gbe_of0]
  gbe0/6 -> [gbe_rxdata]
  gbe0/7 -> [gbe_rxvld]
  gbe0/8 -> [gbe_rxip]
  gbe0/9 -> [gbe_rxport]
  gbe0/10 -> [gbe_rxeof]
  gbe0/11 -> [gbe_rx_bad]
  gbe0/12 -> [gbe_rx_over]
  err_clear_sim4/1 -> gbe_port/1
  gbe_port/1 -> Delay36/1
  err_clear_sim3/1 -> gbe_ip0/1
  gbe_ip0/1 -> Delay37/1
  Delay12/1 -> [eq0_dv]
  [eq0_dv] -> Delay45/1
  arm11/1 -> [fine_tvg_en]
  fine/4(data_index) -> Delay21/1
  katadc0/5(or0) -> [adc_or0]
  katadc0/10(or1) -> [adc_or1]
  katadc0/11(sync0) -> bus_create7/1(in1)
  katadc0/12(sync1) -> bus_create7/2(in2)
  katadc0/13(sync2) -> bus_create7/3(in3)
  katadc0/14(sync3) -> bus_create7/4(in4)
  katadc0/15(data_valid) -> Terminator3/1
  ? -> katadc0/1(sim_data0)
  ? -> katadc0/2(sim_data1)
  ? -> katadc0/3(sim_sync)
  Constant/1 -> katadc0/4(sim_data_valid)
  calc_adc_sum_sq/1(sum_sq) -> adc_sum_sq0/1
  decat0/1(Out1) -> calc_adc_sum_sq/1(In1)
  decat0/2(Out2) -> calc_adc_sum_sq/2(In2)
  decat0/3(Out3) -> calc_adc_sum_sq/3(In3)
  decat0/4(Out4) -> calc_adc_sum_sq/4(In4)
  [adc0] -> decat0/1(In1)
  adc_sum_sq0/1 -> Terminator/1
  [adc1] -> decat1/1(In1)
  calc_adc_sum_sq1/1(sum_sq) -> adc_sum_sq1/1
  decat1/1(Out1) -> calc_adc_sum_sq1/1(In1)
  decat1/2(Out2) -> calc_adc_sum_sq1/2(In2)
  decat1/3(Out3) -> calc_adc_sum_sq1/3(In3)
  decat1/4(Out4) -> calc_adc_sum_sq1/4(In4)
  adc_sum_sq1/1 -> Terminator25/1
  katadc0/1(data0_0) -> bus_create9/1(in1)
  katadc0/2(data0_1) -> bus_create9/2(in2)
  katadc0/3(data0_2) -> bus_create9/3(in3)
  katadc0/4(data0_3) -> bus_create9/4(in4)
  katadc0/6(data1_0) -> bus_create2/1(in1)
  katadc0/7(data1_1) -> bus_create2/2(in2)
  katadc0/8(data1_2) -> bus_create2/3(in3)
  katadc0/9(data1_3) -> bus_create2/4(in4)
  bus_create9/1(bus_out) -> [adc0]
  bus_create2/1(bus_out) -> [adc1]
  fdfs/3(dv_out) -> Delay12/1, Counter8/2
  fdfs/2(data_out) -> Delay8/1
  fdfs/1(sync_out) -> Counter8/1, Delay1/1
  Delay22/1 -> fine/1(sync)
  Delay24/1 -> fine/2(data)
  Slice21/1 -> [coarse_chan_select]
  fine/7(snap_128bit) -> [debug_fine_128]
  fine_ctrl/1 -> Delay13/1
  Constant8/1 -> eq1/2(data_in)
  Constant24/1 -> eq1/3(we)
  eq0/1(data_out) -> bus_create11/1(in1)
  bus_create11/1(bus_out) -> [eq0_coeffs]
  eq1/1(data_out) -> bus_create11/2(in2)
  [gbe_up] -> Subsystem1/5(link_up)
  [gbe_tx] -> Subsystem1/6(led_tx)
  [gbe_txd] -> Subsystem1/1(data_in)
  [gbe_txvld] -> Subsystem1/2(valid_in)
  [gbe_txip] -> Subsystem1/3(ip_in)
  [gbe_txeof] -> Subsystem1/4(eof_in)
  [gbe_tx_full] -> Subsystem1/7(tx_full)
  [gbe_tx_over] -> Subsystem1/8(tx_over)
  [xaui_data] -> Subsystem2/1(data_in)
  [xaui_oob] -> Subsystem2/2(oob_in)
  [xaui_valid] -> Subsystem2/3(we_in)
  [xaui_link_dn] -> Subsystem2/4(link_down)
  arm10/1 -> [adc_protect_disable]
  Constant27/1 -> adc_ctrl0/1
  adc_ctrl0/1 -> Delay39/1
  Constant48/1 -> adc_ctrl1/1
  adc_ctrl1/1 -> Delay40/1
  [adc_bad_latch0] -> Inverter1/1
  Inverter1/1 -> Logical6/1
  [adc_protect_disable] -> Logical6/2
  Logical8/1 -> [adc_en0], katadc0/5(en0)
  Logical6/1 -> Logical8/1
  Slice29/1 -> Logical8/2
  Slice30/1 -> katadc0/6(atten0)
  [adc_bad_latch1] -> Inverter2/1
  Inverter2/1 -> Logical9/1
  [adc_protect_disable] -> Logical9/2
  Logical9/1 -> Logical10/1
  Slice33/1 -> Logical10/2
  Logical10/1 -> [adc_en1], katadc0/7(en1)
  Slice34/1 -> katadc0/8(atten1)
  [adc_en0] -> Inverter5/1
  Subsystem/2(adc0_bad_latch) -> [adc_bad_latch0]
  [adc_sync0] -> Logical5/2
  timing/2(sync) -> [sync]
  Logical5/1 -> timing/4(pps_in), [pps]
  Concat/1 -> timing/2(data_in)
  timing/1(armed) -> Logical14/2, [armed]
  Logical14/1 -> [mrst]
  [sys_rst] -> Logical14/1
  [man_sync] -> Logical5/1
  [arm] -> timing/1(arm)
  sync_period_constant/1 -> timing/3(sync_period)
  Logical1/1 -> edge_detect1/1
  edge_detect1/1 -> [adc_sync0]
  Slice35/1 -> Logical1/1
  Slice36/1 -> Logical1/2
  Slice40/1 -> Logical1/3
  Slice45/1 -> Logical1/4
  [sync_raw0] -> Slice35/1, Slice45/1, Slice40/1, Slice36/1
  [sync_raw0] -> Register3/1
  [adc_sync0] -> Logical11/1
  Logical11/1 -> Register3/2
  [mrst] -> Logical11/2
  Register3/1 -> convert/1(in)
  convert/1(Out1) -> [sync_val]
  [adc0] -> Concat/2
  [adc1] -> Concat/3
  [adc_sync0] -> Concat/1
  timing/3(data_out) -> bus_expand6/1(bus_in)
  Counter1/1 -> Register19/1
  Register19/1 -> Relational/1, Relational1/1, clk_frequency/1
  clk_frequency/1 -> Terminator4/1
  pps_count/1 -> Terminator5/1
  [mrst] -> Counter3/1
  [armed] -> Concat21/1
  Counter3/1 -> Concat21/2
  Concat21/1 -> pps_count/1
  [pps] -> Counter1/1, Counter3/2, Register19/2
  Constant5/1 -> Relational/2
  Constant37/1 -> Relational1/2
  Relational/1 -> Logical21/1
  Relational1/1 -> Logical21/2
  Logical21/1 -> [clk_bad]
  [clr_status] -> Subsystem/1(clr)
  fstatcbits0/1 -> Subsystem/2(coarse_bits)
  fstatfbits0/1 -> Subsystem/3(fine_bits)
  [sync_val] -> Subsystem/4(sync_val)
  [gbe_ldn0] -> Subsystem/5(xuai_ldn)
  [gbe_of0] -> Subsystem/6(xaui_of)
  [clk_bad] -> Subsystem/7(clk_err)
  Inverter5/1 -> Subsystem/8(adc_disabled)
  [qdr_error] -> Subsystem/9(ct_err)
  [adc_or0] -> Subsystem/10(adcOR)
  [fine_fft_or0] -> Subsystem/11(fineFFTOR)
  [crs_fft_or0] -> Subsystem/12(coarseFFTOR)
  [quant_or] -> Subsystem/13(quantOR)
  bus_create7/1(bus_out) -> [sync_raw0]
  fstatus1/1 -> Terminator6/1
  Subsystem3/1(status) -> fstatus1/1
  [adc_en1] -> Inverter3/1
  Subsystem3/2(adc0_bad_latch) -> [adc_bad_latch1]
  [clr_status] -> Subsystem3/1(clr)
  fstatcbits1/1 -> Subsystem3/2(coarse_bits)
  [sync_val] -> Subsystem3/4(sync_val)
  [gbe_ldn0] -> Subsystem3/5(xuai_ldn)
  [gbe_of0] -> Subsystem3/6(xaui_of)
  [clk_bad] -> Subsystem3/7(clk_err)
  Inverter3/1 -> Subsystem3/8(adc_disabled)
  [qdr_error] -> Subsystem3/9(ct_err)
  [adc_or1] -> Subsystem3/10(adcOR)
  [fine_fft_or1] -> Subsystem3/11(fineFFTOR)
  [crs_fft_or1] -> Subsystem3/12(coarseFFTOR)
  [quant_or] -> Subsystem3/13(quantOR)
  Logical7/1 -> leds/1(warning)
  [sync] -> leds/4(sync_led)
  Logical4/1 -> leds/6(comms)
  [pps] -> leds/5(pps)
  [mrst] -> leds/3(rst)
  [fancy_en] -> leds/2(fancy_en)
  [gbe_ldn0] -> Logical4/1
  [gbe_of0] -> Logical4/2
  [adc_en0] -> Inverter4/1
  [adc_en1] -> Inverter6/1
  [adc_or0] -> Logical17/1
  [crs_fft_or0] -> Logical17/2
  Logical17/1 -> leds/9(or0)
  [adc_en0] -> leds/7(adc_en0)
  [adc_en1] -> leds/8(adc_en1)
  [gbe_of0] -> Logical7/2
  [gbe_ldn0] -> Logical7/1
  Inverter4/1 -> Logical7/3
  Inverter6/1 -> Logical7/4
  [clk_bad] -> Logical7/5
  arm12/1 -> [fancy_en]
  repack_for_snap/1(snap_16bit) -> [debug_quant_16]
  Slice24/1 -> [fine_fft_shift]
  qdr_ct/4(snap64) -> [debug_ct_64]
  Delay16/1 -> fdfs/2(sync)
  Delay21/1 -> fdfs/6(index)
  packetiser/3(out_oob) -> [xaui_oob]
  packetiser/2(out_valid) -> [xaui_valid]
  Subsystem4/1(data) -> snap_debug/1(din)
  Subsystem4/2(valid) -> snap_debug/2(we)
  Subsystem4/3(sync) -> snap_debug/3(trig)
  [debug_xaui_128] -> Subsystem4/6(xaui_128)
  [debug_gbetx0_128] -> Subsystem4/7(gbetx0_128)
  Subsystem2/1(debug_out) -> [debug_xaui_128]
  Subsystem1/1(debug_out) -> [debug_gbetx0_128]
  [debug_snap_select] -> Subsystem4/1(select)
  [debug_coarse_72] -> Subsystem4/2(coarse_72)
  [debug_fine_128] -> Subsystem4/3(fine_128)
  [debug_quant_16] -> Subsystem4/4(quant_16)
  [debug_ct_64] -> Subsystem4/5(ct_64)
  arm14/1 -> [debug_snap_select]
  [coarse_chan_select] -> coarse/5(channel_select)
  coarse/4(fft_of1) -> [crs_fft_or1]
  [tvg_en] -> Register2/2
  [ct_tvg] -> Register2/1
  quantisation/1(sync_out) -> ct_tvg/1(syncin)
  quantisation/2(quant_data) -> ct_tvg/2(datain)
  quantisation/3(quant_dv) -> ct_tvg/3(validin)
  Register2/1 -> ct_tvg/4(tvg_en)
  ct_tvg/1(syncout) -> qdr_ct/1(sync), repack_for_snap/1(sync_in)
  ct_tvg/2(dataout) -> qdr_ct/2(d), repack_for_snap/2(data_in)
  ct_tvg/3(validout) -> qdr_ct/3(en), repack_for_snap/3(dv_in)
  packetiser_tvg_contiguous/1(sync_out) -> packetiser/1(sync)
  packetiser_tvg_contiguous/2(dv_out) -> packetiser/2(dv)
  packetiser_tvg_contiguous/3(dout) -> packetiser/3(data)
  qdr_ct/1(sync_out) -> packetiser_tvg_contiguous/1(sync)
  qdr_ct/3(dv) -> packetiser_tvg_contiguous/2(dv)
  qdr_ct/2(q) -> packetiser_tvg_contiguous/3(din)
  Register1/1 -> packetiser_tvg_contiguous/4(use_tvg)
  [mrst] -> fine/6(mrst)
  [tvg_en] -> Register4/2
  [fine_tvg_en] -> Register4/1
  Register4/1 -> fine/5(tvg_en)
  qdr_ct/5(qdr_error) -> [qdr_error]
  fine/1(sync_out) -> Delay16/1
  Delay15/1 -> fdfs/5(dv)
  mcount_msw/1 -> Terminator12/1
  mcount_lsw/1 -> Terminator13/1
  Slice/1 -> mcount_lsw/1
  Slice9/1 -> mcount_msw/1
  [cd_local_time] -> Slice9/1, Slice/1
  edge_detect2/1(out) -> Delay6/1
  Delay6/1 -> [load_now]
  [mrst] -> cd_local_time/1(reset), edge_detect2/1(in)
  [sync] -> cd_local_time/2(sync)
  cd_local_time/1(time) -> [cd_local_time]
  Constant33/1 -> ld_time_msw0/1
  Constant29/1 -> ld_time_lsw0/1
  ld_time_msw0/1 -> Delay18/1
  Slice73/1 -> Concat9/1
  ld_time_lsw0/1 -> Delay19/1
  Constant32/1 -> coarse_delay0/1
  Constant22/1 -> a0_fd0/1
  Constant13/1 -> a1_fd0/1
  a0_fd0/1 -> Delay20/1
  Slice4/1 -> Concat22/4
  Slice7/1 -> Concat22/5
  coarse_delay0/1 -> Delay25/1
  Slice2/1 -> Concat22/1
  Slice3/1 -> Concat22/2
  Slice38/1 -> AddSub/1
  AddSub/1 -> Concat22/3
  Slice13/1 -> [arm0]
  Concat9/1 -> [ld_time0]
  Concat22/1 -> [ld_val0]
  a1_fd0/1 -> Delay26/1
  Constant11/1 -> ld_time_msw1/1
  Constant7/1 -> ld_time_lsw1/1
  ld_time_msw1/1 -> Delay27/1
  Slice12/1 -> Concat2/1
  ld_time_lsw1/1 -> Delay28/1
  Constant10/1 -> coarse_delay1/1
  Constant21/1 -> a0_fd1/1
  Constant16/1 -> a1_fd1/1
  a0_fd1/1 -> Delay29/1
  Slice15/1 -> Concat1/4
  Slice10/1 -> Concat1/5
  coarse_delay1/1 -> Delay30/1
  Slice1/1 -> Concat1/1
  Slice8/1 -> Concat1/2
  Slice14/1 -> AddSub1/1
  AddSub1/1 -> Concat1/3
  Slice11/1 -> [arm1]
  Concat2/1 -> [ld_time1]
  Concat1/1 -> [ld_val1]
  a1_fd1/1 -> Delay32/1
  [sync_val] -> AddSub/2, AddSub1/2
  coarse/5(snap72) -> [debug_coarse_72]
  [cdebug_pol_sel] -> coarse/6(debug_polsel)
  [mrst] -> coarse_delay/1(mrst)
  [sync] -> coarse_delay/2(sync)
  [cd_local_time] -> coarse_delay/3(cd_lt)
  [load_now] -> coarse_delay/4(load_now)
  [data_adc0] -> coarse_delay/5(data0)
  [arm0] -> coarse_delay/6(arm0)
  [ld_time0] -> coarse_delay/7(ld_time0)
  [ld_val0] -> coarse_delay/8(ld_val0)
  [data_adc1] -> coarse_delay/9(data1)
  [arm1] -> coarse_delay/10(arm1)
  [ld_time1] -> coarse_delay/11(ld_time1)
  [ld_val1] -> coarse_delay/12(ld_val1)
  [mrst] -> fdfs/1(mrst)
  edge_detect3/1 -> fdfs/4(window_start)
  Delay14/1 -> fdfs/3(data)
  [fd_fs_tvg] -> Register5/1
  [tvg_en] -> Register5/2
  delay_tr_status0/1(sim_reg_out) -> Terminator17/1
  [arm0] -> fdfs/7(arm0)
  [ld_time0] -> fdfs/8(ld_time0)
  [ld_val0] -> fdfs/9(ld_val0)
  [arm1] -> fdfs/10(arm1)
  [ld_time1] -> fdfs/11(ld_time1)
  [ld_val1] -> fdfs/12(ld_val1)
  Register5/1 -> fdfs/14(tvg_en)
  fine/2(data_out) -> Delay14/1
  fine/3(fft_dv) -> Delay15/1, edge_detect3/1
  fdfs/4(fd_status0) -> delay_tr_status0/1(reg_out)
  delay_tr_status1/1(sim_reg_out) -> Terminator1/1
  fdfs/5(fd_status1) -> delay_tr_status1/1(reg_out)
  [load_now] -> fdfs/13(load_now)
  bus_expand6/1(msb_out3) -> [timing_pps]
  bus_expand6/2(out2) -> [data_adc0]
  bus_expand6/3(lsb_out1) -> [data_adc1]
  Constant25/1 -> trig_level/1
  trig_level/1 -> Delay35/1
  [data_adc1] -> trig1/2(adc_data)
  trig1/3(trig) -> [trig_adc1]
  trig1/2(data) -> [trig_data1]
  [trig_data0] -> adc_snap0/1(din)
  trig0/2(data) -> [trig_data0]
  trig0/3(trig) -> [trig_adc0]
  [sync] -> trig1/1(synci)
  [data_adc0] -> trig0/2(adc_data)
  trig1/1(synco) -> Terminator14/1
  Constant23/1 -> adc_snap0/2(we)
  [trig_sync] -> adc_snap0/3(trig)
  [trig_adc0] -> adc_snap0/4(stop)
  [timing_pps] -> Concat6/1
  [cd_local_time] -> Slice16/1
  Concat6/1 -> trig0/1(synci)
  trig0/1(synco) -> bus_expand/1(bus_in)
  bus_expand/1(msb_out2) -> [trig_sync]
  Slice16/1 -> Concat6/2
  bus_expand/2(lsb_out1) -> [timestamp]
  [timestamp] -> adc_snap0/5(vin)
  [trig_data1] -> adc_snap1/1(din)
  [trig_adc1] -> adc_snap1/4(stop)
  [timestamp] -> adc_snap1/5(vin)
  [trig_sync] -> adc_snap1/3(trig)
  Constant15/1 -> adc_snap1/2(we)
  arm13/1 -> Terminator15/1
  Slice17/1 -> [cdebug_pol_sel]
  Slice18/1 -> [cdebug_chan_sel]
  Slice19/1 -> [cdebug_chan]
  [cdebug_chan_sel] -> coarse/7(debug_chansel)
  [cdebug_chan] -> coarse/8(debug_chan)
  [debug_buffer_72] -> Subsystem4/8(buffer_72)
  [debug_finepfb_72] -> Subsystem4/9(finepfb_72)
  fine/8(snap_buffer72) -> [debug_buffer_72]
  fine/9(snap_pfb72) -> [debug_finepfb_72]
  coarse_delay/1(sync_out) -> coarse/1(sync)
  fine/6(fft_or1) -> [fine_fft_or1]
  coarse_delay/2(data4_0) -> coarse/2(data0)
  coarse_delay/3(data4_1) -> coarse/3(data1)
  [fine_fft_or0] -> Logical17/3
  [adc_or1] -> Logical12/1
  [crs_fft_or1] -> Logical12/2
  [fine_fft_or1] -> Logical12/3
  Logical12/1 -> leds/10(or1)
  [qdr_error] -> Logical7/6
  Delay13/1 -> Slice24/1
  Delay17/1 -> Slice6/1, Slice21/1, Slice17/1, Slice18/1, Slice19/1
  Delay18/1 -> Slice73/1, Slice13/1
  Delay19/1 -> Concat9/2
  Delay20/1 -> Slice3/1, Slice2/1
  Delay25/1 -> Slice38/1
  Delay26/1 -> Slice4/1, Slice7/1
  Delay27/1 -> Slice11/1, Slice12/1
  Delay28/1 -> Concat2/2
  Delay29/1 -> Slice1/1, Slice8/1
  Delay30/1 -> Slice14/1
  Delay32/1 -> Slice10/1, Slice15/1
  Delay35/1 -> trig0/3(trig_pnt), trig1/3(trig_pnt)
  Delay36/1 -> [gbe_txport]
  Delay37/1 -> [gbe_base_ip]
  Delay39/1 -> Slice29/1, Slice30/1
  Delay40/1 -> Slice34/1, Slice33/1
  Delay41/1 -> Slice78/1, man_sync1/1, arm1/1, arm2/1, arm9/1, arm10/1, arm7/1, arm11/1, arm13/1, arm14/1, arm6/1, arm5/1, arm4/1, arm3/1, arm12/1, arm8/1
  Delay42/1 -> [board_id]
  Delay43/1 -> quantisation/1(sync)
  Delay44/1 -> quantisation/2(data)
  Delay45/1 -> quantisation/3(dv)
  Delay46/1 -> quantisation/4(eq_bus)
  fstatfbits1/1 -> Subsystem3/3(fine_bits)
